simulink model "untitled"  (Simulink 8.7)
settings: Solver=VariableStepAuto  StartTime=0.0  StopTime=179.9  RelTol=1e-3
values from neighbouring files (symbols this model uses):
  u_stat = [0;100;200;250;300;350;400;450;500;550;600;700;750]    [Untitled.m]    (also in ident.mat = [0 100 200 300 400 500 600 700])
  y_stat = y_stat*K    [Sebessegszabalyozas_sim.m]    (also in Untitled.m = [0;  0;  0;  0; 42; 67; 80; 95;110;120;130;160;170]; ident.mat = [0 0 0 32 100 160 216 260])
settings Model: Creator=Mester Ádám  LastModifiedBy=Mester Ádám
settings DataIOCC: LimitDataPoints=off  SaveFormat=Dataset
settings DebuggingCC: UnderspecifiedInitializationDetection=Simplified  MergeDetectMultiDrivingBlocksExec=error
settings HardwareCC: ProdBitPerPointer=64  ProdLargestAtomicFloat=Float  ProdIntDivRoundTo=Zero  ProdEndianess=LittleEndian  ProdWordSize=64  ProdHWDeviceType=Intel->x86-64 (Windows64)
settings ModelReferenceCC: PropagateSignalLabelsOutOfModel=on
settings ConfigComp: CovModelRefEnable=off

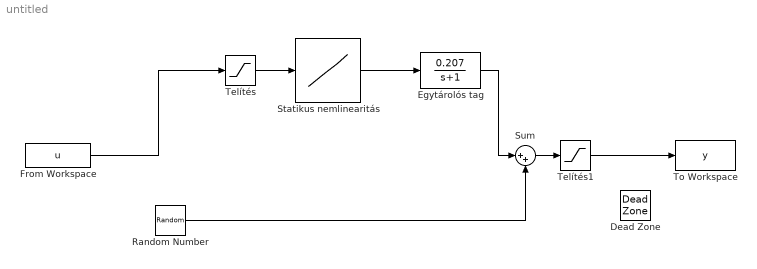
== system untitled ==
  Dead Zone : DeadZone  LowerValue=-20  UpperValue=20  SaturateOnIntegerOverflow=on
  Egytárolós tag : TransferFcn  Numerator=[0.207]  Denominator=[1 1]
  From Workspace : FromWorkspace  VariableName=u  SampleTime=0.1
  Random Number : RandomNumber  Variance=20  SampleTime=0.1
  Statikus nemlinearitás : Lookup_n-D  NumberOfTableDimensions=1  BreakpointsForDimension1=u_stat  Table=y_stat/0.207  InternalRulePriority=Speed  RndMeth=Simplest  InputSameDT=on
  Sum : Sum  Inputs=|++
  Telítés : Saturate  UpperLimit=180/0.207  LowerLimit=0
  Telítés1 : Saturate  UpperLimit=inf  LowerLimit=0
  To Workspace : ToWorkspace  VariableName=y  SaveFormat=Structure  SampleTime=0.1
  wires:
  Random Number/1 -> Sum/2
  Egytárolós tag/1 -> Sum/1
  From Workspace/1 -> Telítés/1
  Telítés/1 -> Statikus nemlinearitás/1
  Statikus nemlinearitás/1 -> Egytárolós tag/1
  Sum/1 -> Telítés1/1
  Telítés1/1 -> To Workspace/1
